simulink model "cw6_model_Gajda"  (R2017b)
settings: Solver=VariableStepAuto  StartTime=0.0  StopTime=500.0  MaxStep=0.01  MinStep=0.001  RelTol=1e-6
values from neighbouring files (symbols this model uses):
  A = [-a0 a0; b0 (-b0-b1)]    [cw6_dane_Gajda.m]
  a0 = 1/(R1*C1)    (= 0.2)    [cw6_dane_Gajda.m]
  a1 = 1/C1    (= 0.1)    [cw6_dane_Gajda.m]
  B = [a1; 0]    [cw6_dane_Gajda.m]
  b0 = 1/(R1*C2)    (= 0.4)    [cw6_dane_Gajda.m]
  b1 = 1/(R2*C2)    (= 0.1)    [cw6_dane_Gajda.m]
  C = [0 1]    [cw6_dane_Gajda.m]
  D = [0]    [cw6_dane_Gajda.m]
settings Model: Creator=MG  LastModifiedBy=MG
settings DataIOCC: SaveFormat=Array

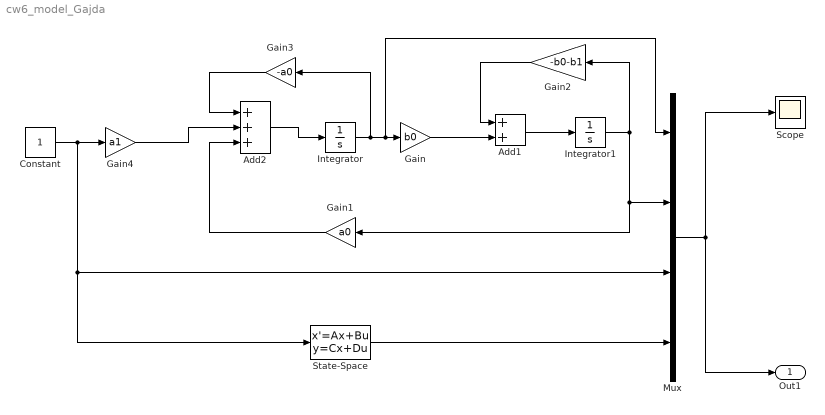
== system cw6_model_Gajda ==
  Add1 : Sum
  Add2 : Sum  Inputs=+++
  Constant : Constant
  Gain : Gain  Gain=b0
  Gain1 : Gain  Gain=a0
  Gain2 : Gain  Gain=-b0-b1
  Gain3 : Gain  Gain=-a0
  Gain4 : Gain  Gain=a1
  Integrator : Integrator
  Integrator1 : Integrator
  Mux : Mux
  Scope : Scope
  State-Space : StateSpace  A=A  B=B  C=C  D=D  InitialCondition=0
  Out1 : Outport  VectorParamsAs1DForOutWhenUnconnected=on
  wires:
  Gain1/1 -> Add2/3
  Integrator/1 -> Gain3/1, Mux/1, Gain/1
  Constant/1 -> State-Space/1, Mux/3, Gain4/1
  Gain/1 -> Add1/2
  Gain2/1 -> Add1/1
  Add2/1 -> Integrator/1
  Integrator1/1 -> Gain1/1, Mux/2, Gain2/1
  Gain4/1 -> Add2/2
  Gain3/1 -> Add2/1
  Mux/1 -> Scope/1, Out1/1
  Add1/1 -> Integrator1/1
  State-Space/1 -> Mux/4
